simulink model "asbdhc2(1)"  (R2024b)
settings: Solver=ode23  StartTime=0.0  StopTime=100  MaxStep=1/30  RelTol=1e-2  AbsTol=1e-3  EnableMultiTasking=on
PreLoadFcn:
  | load asbdhc2_init;
model workspace (MAT data in the model file):
  op_trim1 : opcond.OperatingReport (value not decoded)
  op_trim2 : opcond.OperatingReport (value not decoded)
  op_trim3 : opcond.OperatingReport (value not decoded)
values from neighbouring files (symbols this model uses):
  beaver_b = 14.63    [aero.mat]
  beaver_c = 1.5875    [aero.mat]
  beaver_init_p = 0    [aero.mat]
  beaver_init_q = 0    [aero.mat]
  beaver_init_r = 0    [aero.mat]
  beaver_init_roll = 0    [aero.mat]
  beaver_mass = 2288.231    [aero.mat]
  Cl_alpha2_dpt = -0.01406    [aero.mat]
  Cl_beta = -0.0618    [aero.mat]
  Cl_da = -0.09917    [aero.mat]
  Cl_da_alpha = -0.08269    [aero.mat]
  Cl_dr = 0.006934    [aero.mat]
  Cl_p = -0.5045    [aero.mat]
  Cl_r = 0.1695    [aero.mat]
  Cm0 = 0.09448    [aero.mat]
  Cm_alpha = -0.6028    [aero.mat]
  Cm_alpha2 = -2.14    [aero.mat]
  Cm_beta2 = 0.6921    [aero.mat]
  Cm_de = -1.921    [aero.mat]
  Cm_df = 0.4072    [aero.mat]
  Cm_dpt = -0.07895    [aero.mat]
  Cm_q = -15.56    [aero.mat]
  Cm_r = -0.3118    [aero.mat]
  Cn_beta = 0.006719    [aero.mat]
  Cn_beta3 = 0.1373    [aero.mat]
  Cn_da = -0.003872    [aero.mat]
  Cn_dpt3 = -0.003026    [aero.mat]
  Cn_dr = -0.08265    [aero.mat]
  Cn_p = -0.1585    [aero.mat]
  Cn_q = 0.1595    [aero.mat]
  Cn_r = -0.1112    [aero.mat]
  Cx0 = -0.03554    [aero.mat]
  Cx_alpha = 0.00292    [aero.mat]
  Cx_alpha2 = 5.459    [aero.mat]
  Cx_alpha3 = -5.162    [aero.mat]
  Cx_df = -0.09447    [aero.mat]
  Cx_df_alpha = 1.106    [aero.mat]
  Cx_dpt = 0.1161    [aero.mat]
  Cx_dpt2_alpha = 0.1453    [aero.mat]
  Cx_dr = 0.03412    [aero.mat]
  Cx_q = -0.6748    [aero.mat]
  Cy0 = -0.002226    [aero.mat]
  Cy_beta = -0.7678    [aero.mat]
  Cy_da = -0.02956    [aero.mat]
  Cy_dr = 0.1158    [aero.mat]
  Cy_dr_alpha = 0.5238    [aero.mat]
  Cy_p = -0.124    [aero.mat]
  Cy_r = 0.3666    [aero.mat]
  Cz0 = -0.05504    [aero.mat]
  Cz_alpha = -5.578    [aero.mat]
  Cz_alpha3 = 3.442    [aero.mat]
  Cz_de = -0.398    [aero.mat]
  Cz_de_beta = -15.93    [aero.mat]
  Cz_df = -1.377    [aero.mat]
  Cz_df_alpha = -1.261    [aero.mat]
  Cz_dpt = -0.1563    [aero.mat]
  Cz_q = -2.988    [aero.mat]
  uaero0 = [-0.0317656979071 -0.0320210159663 -0.0365180369264 0]    [aero.mat]
undefined symbols (not defined in the file or in its folder): Earth, F, Light, MIL, Receive, report2, Send, WGS84
libraries: aerolibconvert2 x3, aerolibwind2 x3, slpidlib x3, aerolibasang x2, aerolibfltsims x2, aerolibanimutils x2, shared6dof x1, aerolibadyn x1, aerolibatmos2 x1, simulink x1, aerolibtransform2 x1
(part 2 of 2)

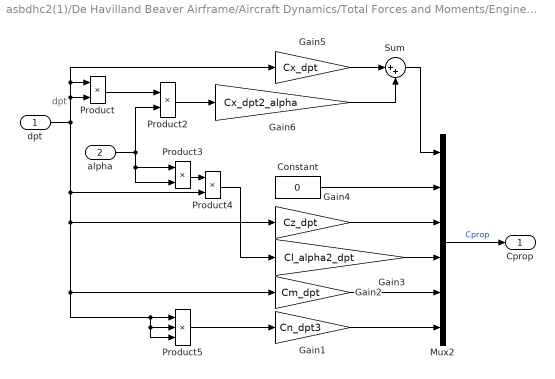
== system asbdhc2(1)/De Havilland Beaver Airframe/Aircraft Dynamics/Total Forces and Moments/Engine /eng ==
  note: dpt
  dpt : Inport
  alpha : Inport  Port=2  Unit=rad
  Constant : Constant  Value=0
  Gain1 : Gain  Gain=Cn_dpt3  SaturateOnIntegerOverflow=on  OutDataTypeStr=Inherit: Same as input  ParamDataTypeStr=Inherit: Same as input
  Gain2 : Gain  Gain=Cm_dpt  SaturateOnIntegerOverflow=on  OutDataTypeStr=Inherit: Same as input  ParamDataTypeStr=Inherit: Same as input
  Gain3 : Gain  Gain=Cl_alpha2_dpt  SaturateOnIntegerOverflow=on  OutDataTypeStr=Inherit: Same as input  ParamDataTypeStr=Inherit: Same as input
  Gain4 : Gain  Gain=Cz_dpt  SaturateOnIntegerOverflow=on  OutDataTypeStr=Inherit: Same as input  ParamDataTypeStr=Inherit: Same as input
  Gain5 : Gain  Gain=Cx_dpt  SaturateOnIntegerOverflow=on  OutDataTypeStr=Inherit: Same as input  ParamDataTypeStr=Inherit: Same as input
  Gain6 : Gain  Gain=Cx_dpt2_alpha  SaturateOnIntegerOverflow=on  OutDataTypeStr=Inherit: Same as input  ParamDataTypeStr=Inherit: Same as input
  Mux2 : Mux  Inputs=6
  Product{,2..4} (4 alike) : Product  SaturateOnIntegerOverflow=on  OutDataTypeStr=Inherit: Same as first input
  Product5 : Product  Inputs=3  SaturateOnIntegerOverflow=on  OutDataTypeStr=Inherit: Same as first input
  Sum : Sum  Inputs=|++  SaturateOnIntegerOverflow=on
  Cprop : Outport  VectorParamsAs1DForOutWhenUnconnected=off
  wires:
  Product5/1 -> Gain1/1
  Sum/1 -> Mux2/1
  Gain6/1 -> Sum/2
  Gain5/1 -> Sum/1
  Constant/1 -> Mux2/2
  Gain4/1 -> Mux2/3
  Gain3/1 -> Mux2/4
  Gain2/1 -> Mux2/5
  Gain1/1 -> Mux2/6
  Product4/1 -> Gain3/1
  Product2/1 -> Gain6/1
  dpt/1 -> Gain5/1, Product/1, Product/2, Product5/3, Product5/2, Product5/1, Gain2/1, Gain4/1, Product4/2
  alpha/1 -> Product2/2, Product3/1, Product3/2
  Mux2/1 -> Cprop/1  "Cprop"
  Product/1 -> Product2/1
  Product3/1 -> Product4/1

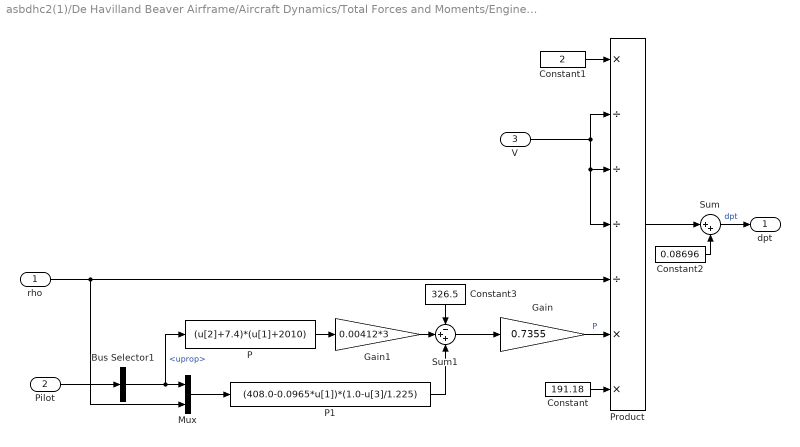
== system asbdhc2(1)/De Havilland Beaver Airframe/Aircraft Dynamics/Total Forces and Moments/Engine /pow ==
  rho : Inport  Unit=kg/m^3
  Pilot : Inport  Port=2
  V : Inport  Port=3  Unit=m/s
  Bus Selector1 : BusSelector  OutputSignals=uprop
  Constant : Constant  Value=191.18
  Constant1 : Constant  Value=2
  Constant2 : Constant  Value=0.08696
  Constant3 : Constant  Value=326.5
  Gain : Gain  Gain=0.7355  SaturateOnIntegerOverflow=on  OutDataTypeStr=Inherit: Same as input  ParamDataTypeStr=Inherit: Same as input
  Gain1 : Gain  Gain=0.00412*3  SaturateOnIntegerOverflow=on  OutDataTypeStr=Inherit: Same as input  ParamDataTypeStr=Inherit: Same as input
  Mux : Mux  Inputs=2
  P : Fcn  Expr=(u[2]+7.4)*(u[1]+2010)
  P1 : Fcn  Expr=(408.0-0.0965*u[1])*(1.0-u[3]/1.225)
  Product : Product  Inputs=*////**  SaturateOnIntegerOverflow=on  OutDataTypeStr=Inherit: Same as first input
  Sum : Sum  Inputs=|++  SaturateOnIntegerOverflow=on
  Sum1 : Sum  Inputs=-++  SaturateOnIntegerOverflow=on
  dpt : Outport  VectorParamsAs1DForOutWhenUnconnected=off
  wires:
  P1/1 -> Sum1/3
  Constant3/1 -> Sum1/1
  Gain1/1 -> Sum1/2
  Mux/1 -> P1/1
  Sum1/1 -> Gain/1
  P/1 -> Gain1/1
  Gain/1 -> Product/6  "P"
  rho/1 -> Mux/2, Product/5
  Sum/1 -> dpt/1  "dpt"
  V/1 -> Product/4, Product/3, Product/2
  Bus Selector1/1 -> P/1, Mux/1  "<uprop>"
  Constant/1 -> Product/7
  Constant1/1 -> Product/1
  Product/1 -> Sum/1
  Constant2/1 -> Sum/2
  Pilot/1 -> Bus Selector1/1

== system asbdhc2(1)/De Havilland Beaver Airframe/Aircraft Dynamics/Total Forces and Moments/Aerodynamics/Actuator Increments/Aileron ==
  alpha : Inport  Unit=rad
  Actuators : Inport  Port=2  Unit=rad
  Gain1 : Gain  Gain=0  SaturateOnIntegerOverflow=on  OutDataTypeStr=Inherit: Same as input  ParamDataTypeStr=Inherit: Same as input
  Gain2 : Gain  Gain=Cy_da  SaturateOnIntegerOverflow=on  OutDataTypeStr=Inherit: Same as input  ParamDataTypeStr=Inherit: Same as input
  Gain3 : Gain  Gain=0  SaturateOnIntegerOverflow=on  OutDataTypeStr=Inherit: Same as input  ParamDataTypeStr=Inherit: Same as input
  Gain4 : Gain  Gain=Cn_da  SaturateOnIntegerOverflow=on  OutDataTypeStr=Inherit: Same as input  ParamDataTypeStr=Inherit: Same as input
  Gain5 : Gain  Gain=0  SaturateOnIntegerOverflow=on  OutDataTypeStr=Inherit: Same as input  ParamDataTypeStr=Inherit: Same as input
  Gain6 : Gain  Gain=Cl_da  SaturateOnIntegerOverflow=on  OutDataTypeStr=Inherit: Same as input  ParamDataTypeStr=Inherit: Same as input
  Gain7 : Gain  Gain=Cl_da_alpha  SaturateOnIntegerOverflow=on  OutDataTypeStr=Inherit: Same as input  ParamDataTypeStr=Inherit: Same as input
  Mux1 : Mux  Inputs=6
  Product4 : Product  InputSameDT=on  SaturateOnIntegerOverflow=on  OutDataTypeStr=Inherit: Same as first input
  Selector1 : Selector  IndexMode=Zero-based  InputPortWidth=4  IndexOptions=Index vector (dialog)  Indices=1  OutputSizes=1
  Sum1 : Sum  Inputs=++|  SaturateOnIntegerOverflow=on
  delCoeff : Outport  VectorParamsAs1DForOutWhenUnconnected=off
  wires:
  Gain6/1 -> Sum1/1
  Sum1/1 -> Mux1/4
  Gain7/1 -> Sum1/2
  Product4/1 -> Gain7/1
  Gain1/1 -> Mux1/1  "Cx"
  alpha/1 -> Product4/2
  Actuators/1 -> Selector1/1
  Mux1/1 -> delCoeff/1
  Gain2/1 -> Mux1/2  "Cy"
  Gain3/1 -> Mux1/3  "Cz"
  Gain5/1 -> Mux1/5  "Cm"
  Gain4/1 -> Mux1/6
  Selector1/1 -> Gain1/1, Gain2/1, Gain3/1, Gain6/1, Product4/1, Gain5/1, Gain4/1

== system asbdhc2(1)/De Havilland Beaver Airframe/Aircraft Dynamics/Total Forces and Moments/Aerodynamics/Actuator Increments/Elevator ==
  Actuators : Inport
  Beta : Inport  Port=2  Unit=rad
  Constant1 : Constant  Value=0
  Gain1 : Gain  Gain=Cz_de  SaturateOnIntegerOverflow=on  OutDataTypeStr=Inherit: Same as input  ParamDataTypeStr=Inherit: Same as input
  Gain2 : Gain  Gain=Cz_de_beta  SaturateOnIntegerOverflow=on  OutDataTypeStr=Inherit: Same as input  ParamDataTypeStr=Inherit: Same as input
  Gain3 : Gain  Gain=Cm_de  SaturateOnIntegerOverflow=on  OutDataTypeStr=Inherit: Same as input  ParamDataTypeStr=Inherit: Same as input
  Mux1 : Mux  Inputs=6
  Product4 : Product  Inputs=3  InputSameDT=on  SaturateOnIntegerOverflow=on  OutDataTypeStr=Inherit: Same as first input
  Selector1 : Selector  IndexMode=Zero-based  InputPortWidth=4  IndexOptions=Index vector (dialog)  Indices=0  OutputSizes=1
  Sum1 : Sum  SaturateOnIntegerOverflow=on
  delCoeff : Outport  VectorParamsAs1DForOutWhenUnconnected=off
  wires:
  Gain3/1 -> Mux1/5
  Gain1/1 -> Sum1/2
  Gain2/1 -> Sum1/1
  Sum1/1 -> Mux1/3
  Product4/1 -> Gain2/1
  Beta/1 -> Product4/2, Product4/1
  Mux1/1 -> delCoeff/1
  Selector1/1 -> Gain3/1, Gain1/1, Product4/3
  Constant1/1 -> Mux1/1, Mux1/2, Mux1/4, Mux1/6
  Actuators/1 -> Selector1/1

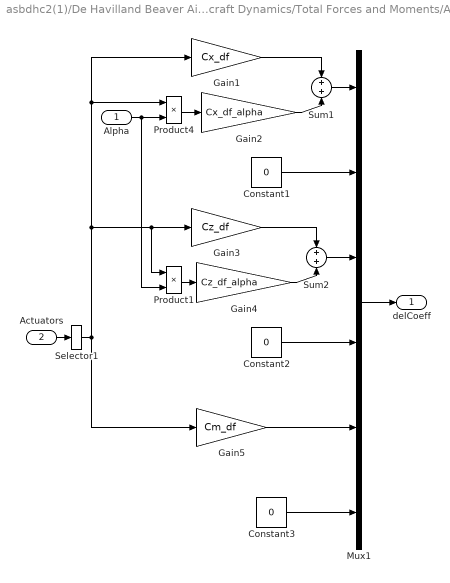
== system asbdhc2(1)/De Havilland Beaver Airframe/Aircraft Dynamics/Total Forces and Moments/Aerodynamics/Actuator Increments/Flap ==
  Alpha : Inport  Unit=rad
  Actuators : Inport  Port=2  Unit=rad
  Constant1 : Constant  Value=0
  Constant2 : Constant  Value=0
  Constant3 : Constant  Value=0
  Gain1 : Gain  Gain=Cx_df  SaturateOnIntegerOverflow=on  OutDataTypeStr=Inherit: Same as input  ParamDataTypeStr=Inherit: Same as input
  Gain2 : Gain  Gain=Cx_df_alpha  SaturateOnIntegerOverflow=on  OutDataTypeStr=Inherit: Same as input  ParamDataTypeStr=Inherit: Same as input
  Gain3 : Gain  Gain=Cz_df  SaturateOnIntegerOverflow=on  OutDataTypeStr=Inherit: Same as input  ParamDataTypeStr=Inherit: Same as input
  Gain4 : Gain  Gain=Cz_df_alpha  SaturateOnIntegerOverflow=on  OutDataTypeStr=Inherit: Same as input  ParamDataTypeStr=Inherit: Same as input
  Gain5 : Gain  Gain=Cm_df  SaturateOnIntegerOverflow=on  OutDataTypeStr=Inherit: Same as input  ParamDataTypeStr=Inherit: Same as input
  Mux1 : Mux  Inputs=6
  Product1 : Product  InputSameDT=on  SaturateOnIntegerOverflow=on  OutDataTypeStr=Inherit: Same as first input
  Product4 : Product  InputSameDT=on  SaturateOnIntegerOverflow=on  OutDataTypeStr=Inherit: Same as first input
  Selector1 : Selector  IndexMode=Zero-based  InputPortWidth=4  IndexOptions=Index vector (dialog)  Indices=3  OutputSizes=1
  Sum1 : Sum  SaturateOnIntegerOverflow=on
  Sum2 : Sum  SaturateOnIntegerOverflow=on
  delCoeff : Outport  VectorParamsAs1DForOutWhenUnconnected=off
  wires:
  Selector1/1 -> Gain1/1, Product4/1, Product1/1, Gain3/1, Gain5/1
  Actuators/1 -> Selector1/1
  Gain5/1 -> Mux1/5
  Gain3/1 -> Sum2/1
  Gain4/1 -> Sum2/2
  Product1/1 -> Gain4/1
  Gain1/1 -> Sum1/1
  Gain2/1 -> Sum1/2
  Product4/1 -> Gain2/1
  Alpha/1 -> Product1/2, Product4/2
  Mux1/1 -> delCoeff/1
  Sum1/1 -> Mux1/1
  Sum2/1 -> Mux1/3
  Constant1/1 -> Mux1/2
  Constant2/1 -> Mux1/4
  Constant3/1 -> Mux1/6

== system asbdhc2(1)/De Havilland Beaver Airframe/Aircraft Dynamics/Total Forces and Moments/Aerodynamics/Actuator Increments/Rudder ==
  Alpha : Inport  Unit=rad
  Actuators : Inport  Port=2  Unit=rad
  Constant1 : Constant  Value=0
  Constant2 : Constant  Value=0
  Gain1 : Gain  Gain=Cl_dr  SaturateOnIntegerOverflow=on  OutDataTypeStr=Inherit: Same as input  ParamDataTypeStr=Inherit: Same as input
  Gain2 : Gain  Gain=Cn_dr  SaturateOnIntegerOverflow=on  OutDataTypeStr=Inherit: Same as input  ParamDataTypeStr=Inherit: Same as input
  Gain3 : Gain  Gain=Cy_dr_alpha  SaturateOnIntegerOverflow=on  OutDataTypeStr=Inherit: Same as input  ParamDataTypeStr=Inherit: Same as input
  Gain4 : Gain  Gain=Cy_dr  SaturateOnIntegerOverflow=on  OutDataTypeStr=Inherit: Same as input  ParamDataTypeStr=Inherit: Same as input
  Gain5 : Gain  Gain=Cx_dr  SaturateOnIntegerOverflow=on  OutDataTypeStr=Inherit: Same as input  ParamDataTypeStr=Inherit: Same as input
  Mux1 : Mux  Inputs=6
  Product1 : Product  InputSameDT=on  SaturateOnIntegerOverflow=on  OutDataTypeStr=Inherit: Same as first input
  Selector1 : Selector  IndexMode=Zero-based  InputPortWidth=4  IndexOptions=Index vector (dialog)  Indices=2  OutputSizes=1
  Sum1 : Sum  SaturateOnIntegerOverflow=on
  delCoeff : Outport  VectorParamsAs1DForOutWhenUnconnected=off
  wires:
  Gain5/1 -> Mux1/1
  Gain4/1 -> Sum1/1
  Gain3/1 -> Sum1/2
  Gain1/1 -> Mux1/4
  Gain2/1 -> Mux1/6
  Product1/1 -> Gain3/1
  Alpha/1 -> Product1/2
  Mux1/1 -> delCoeff/1
  Actuators/1 -> Selector1/1
  Sum1/1 -> Mux1/2
  Constant1/1 -> Mux1/3
  Constant2/1 -> Mux1/5
  Selector1/1 -> Gain5/1, Gain4/1, Product1/1, Gain1/1, Gain2/1

== system asbdhc2(1)/De Havilland Beaver Airframe/Aircraft Dynamics/Total Forces and Moments/Aerodynamics/Body Rate Damping/p ==
  Constant1 : Constant  Value=0
  Constant2 : Constant  Value=Cy_p
  Constant3 : Constant  Value=Cl_p
  Constant4 : Constant  Value=Cn_p
  Mux1 : Mux  Inputs=6
  delCoeff : Outport  VectorParamsAs1DForOutWhenUnconnected=off
  wires:
  Constant2/1 -> Mux1/2
  Mux1/1 -> delCoeff/1
  Constant1/1 -> Mux1/5, Mux1/3, Mux1/1
  Constant4/1 -> Mux1/6
  Constant3/1 -> Mux1/4

== system asbdhc2(1)/De Havilland Beaver Airframe/Aircraft Dynamics/Total Forces and Moments/Aerodynamics/Body Rate Damping/q ==
  Constant1 : Constant  Value=0
  Constant2 : Constant  Value=Cz_q
  Constant3 : Constant  Value=Cx_q
  Constant4 : Constant  Value=Cm_q
  Constant5 : Constant  Value=Cn_q
  Mux1 : Mux  Inputs=6
  delCoeff : Outport  VectorParamsAs1DForOutWhenUnconnected=off
  wires:
  Constant2/1 -> Mux1/3
  Constant5/1 -> Mux1/6
  Constant1/1 -> Mux1/4, Mux1/2
  Constant4/1 -> Mux1/5
  Constant3/1 -> Mux1/1
  Mux1/1 -> delCoeff/1

== system asbdhc2(1)/De Havilland Beaver Airframe/Aircraft Dynamics/Total Forces and Moments/Aerodynamics/Body Rate Damping/r ==
  Constant : Constant  Value=0
  Constant1 : Constant  Value=Cy_r
  Constant2 : Constant  Value=Cl_r
  Constant3 : Constant  Value=Cm_r
  Constant4 : Constant  Value=Cn_r
  Mux1 : Mux  Inputs=6
  delCoeff : Outport  VectorParamsAs1DForOutWhenUnconnected=off
  wires:
  Constant3/1 -> Mux1/5
  Constant1/1 -> Mux1/2
  Constant4/1 -> Mux1/6
  Constant2/1 -> Mux1/4
  Constant/1 -> Mux1/3, Mux1/1
  Mux1/1 -> delCoeff/1

== matlab function asbdhc2(1)/De Havilland Beaver Airframe/Aircraft Dynamics/MATLAB Function ==
  data: Vx input; TAngle output; Vy input; Vz input; Ve_tot output
function [TAngle,Ve_tot] = Track_Angle(Vx,Vy,Vz)

Vh=sqrt(Vx^2+Vy^2);
TAngle=Vz/Vh;
Ve_tot=sqrt(Vx^2+Vy^2+Vz^2);

== matlab function asbdhc2(1)/De Havilland Beaver Airframe/Aircraft Dynamics/MATLAB Function2 ==
  data: Ax input; Abe_tot output; Ay input; Az input
function Abe_tot = Abe_tot_acc(Ax,Ay,Az)

Abe_tot=sqrt(Ax^2+Ay^2+Az^2);
